simulink model "ART_1G_MMU_SLDRT"  (R2021a)
settings: configuration reference "Normal_SLDRT" (kept outside this file)
undefined symbols (not defined in the file): channel, desired_trajectory_index, group_IP_address, receive_multicast_udp_port_initialize, release_receive_multicast_udp_buffer, release_send_multicast_udp_buffer, send_multicast_udp_data, send_multicast_udp_port_initialize, TRDP_COM_ID_MC2_IDS2MMU, TRDP_COM_ID_MC2_MMU2IDS_POINT, TRDP_COM_ID_MC2_MMU2IDS_SEGMENT, TRDP_CONFIG_MC2_IDS2MMU, TRDP_output, TRDP_SIGNALS_MC2_IDS2MMU, TRDP_SIGNALS_MC2_MMU2IDS_POINT, TRDP_SIGNALS_MC2_MMU2IDS_SEGMENT, UDP_port
libraries: etargetslib x2, simulink x1, sldrtlib x1
settings Model: DataDictionary=ART_1G_MMU.sldd  Creator=xinrui  LastModifiedBy=xinrui
settings ConfigSetRef: SourceName=Normal_SLDRT

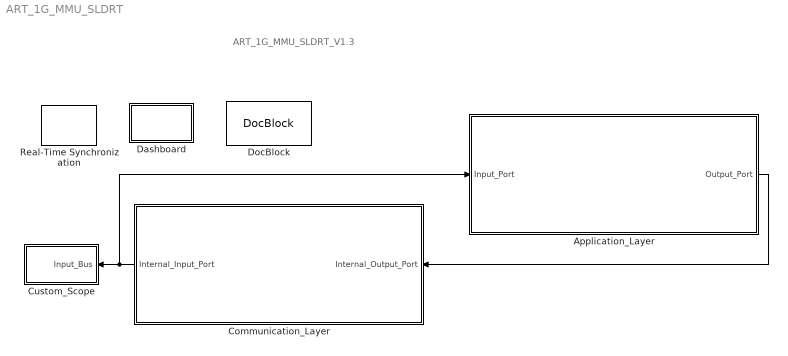
== system ART_1G_MMU_SLDRT ==
  note: ART_1G_MMU_SLDRT_V1.3
  Application_Layer : Subsystem
  Communication_Layer : Subsystem
  Custom_Scope : Subsystem
  Dashboard : Subsystem
  DocBlock : simulink/Model-Wide Utilities/DocBlock  DocumentType=HTML  mask(DocBlock){}
      mask Display:
      | plot([.8 0 0 1 1 .8 .8 1],[1 1 0 0 .8 1 .8 .8]);
      | text(.5,.6,'CHANGELOG','horizontalalignment','center');
      | text(.95,.05,get_param(gcb,'DocumentType'),'verticalalignment','bottom','horizontalalignment','right');
  Real-Time Synchronization : sldrtlib/Real-Time Synchronization  SampleTime=-1  MaxMissedTicks=10  ShowMissedTicks=off  YieldWhenWaiting=off
  wires:
  Application_Layer/1(Output_Port) -> Communication_Layer/1(Internal_Output_Port)
  Communication_Layer/1(Internal_Input_Port) -> Custom_Scope/1(Input_Bus), Application_Layer/1(Input_Port)

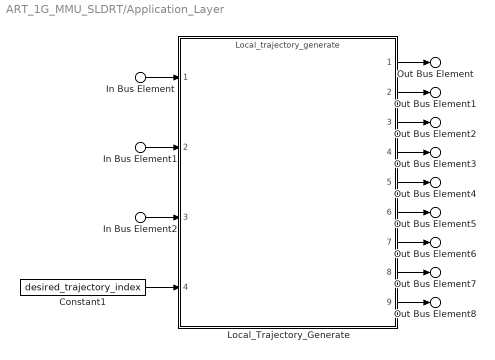
== system ART_1G_MMU_SLDRT/Application_Layer ==
  In Bus Element : Inport  PortName=Input_Port  Element=GNSS_info.ENU_yaw_angle
  In Bus Element1 : Inport  PortName=Input_Port  Element=GNSS_info.ENU_x
  In Bus Element2 : Inport  PortName=Input_Port  Element=GNSS_info.ENU_y
  Constant1 : Constant  Value=desired_trajectory_index  OutDataTypeStr=int8  SampleTime=-1
  Local_Trajectory_Generate : ModelReference  ModelNameDialog=Local_trajectory_generate.slx  SimulationMode=Normal  ModelReferenceVersion=1.197
  Out Bus Element : Outport  PortName=Output_Port  Element=reference_trajectory_info.way_point_number
  Out Bus Element1 : Outport  PortName=Output_Port  Element=reference_trajectory_info.trajectory_yaw_angle
  Out Bus Element2 : Outport  PortName=Output_Port  Element=reference_trajectory_info.trajectory_x
  Out Bus Element3 : Outport  PortName=Output_Port  Element=reference_trajectory_info.trajectory_y
  Out Bus Element4 : Outport  PortName=Output_Port  Element=reference_trajectory_info.trajectory_curvature
  Out Bus Element5 : Outport  PortName=Output_Port  Element=reference_trajectory_info.segment_length
  Out Bus Element6 : Outport  PortName=Output_Port  Element=reference_trajectory_info.segment_ID
  Out Bus Element7 : Outport  PortName=Output_Port  Element=reference_trajectory_info.vision_priority
  Out Bus Element8 : Outport  PortName=Output_Port  Element=reference_trajectory_info.GNSS_priority
  wires:
  In Bus Element/1 -> Local_Trajectory_Generate/1
  In Bus Element1/1 -> Local_Trajectory_Generate/2
  In Bus Element2/1 -> Local_Trajectory_Generate/3
  Constant1/1 -> Local_Trajectory_Generate/4
  Local_Trajectory_Generate/1 -> Out Bus Element/1
  Local_Trajectory_Generate/2 -> Out Bus Element1/1
  Local_Trajectory_Generate/3 -> Out Bus Element2/1
  Local_Trajectory_Generate/4 -> Out Bus Element3/1
  Local_Trajectory_Generate/5 -> Out Bus Element4/1
  Local_Trajectory_Generate/6 -> Out Bus Element5/1
  Local_Trajectory_Generate/7 -> Out Bus Element6/1
  Local_Trajectory_Generate/8 -> Out Bus Element7/1
  Local_Trajectory_Generate/9 -> Out Bus Element8/1

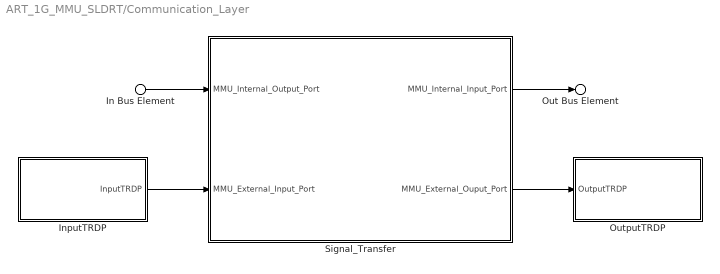
== system ART_1G_MMU_SLDRT/Communication_Layer ==
  In Bus Element : Inport  PortName=Internal_Output_Port
  InputTRDP : Subsystem
  OutputTRDP : Subsystem
  Signal_Transfer : Subsystem
  Out Bus Element : Outport  PortName=Internal_Input_Port
  wires:
  InputTRDP/1(InputTRDP) -> Signal_Transfer/2(MMU_External_Input_Port)
  Signal_Transfer/2(MMU_External_Ouput_Port) -> OutputTRDP/1(OutputTRDP)
  Signal_Transfer/1(MMU_Internal_Input_Port) -> Out Bus Element/1
  In Bus Element/1 -> Signal_Transfer/1(MMU_Internal_Output_Port)

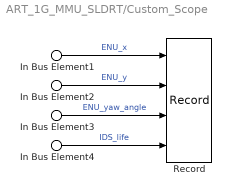
== system ART_1G_MMU_SLDRT/Custom_Scope ==
  In Bus Element4 : Inport  PortName=Input_Bus  Element=GNSS_info.IDS_life
  In Bus Element3 : Inport  PortName=Input_Bus  Element=GNSS_info.ENU_yaw_angle
  In Bus Element1 : Inport  PortName=Input_Bus  Element=GNSS_info.ENU_x
  In Bus Element2 : Inport  PortName=Input_Bus  Element=GNSS_info.ENU_y
  Record : Record  FileSettingsInternal="{\"entries\":[{\"content\":{\"excelSettings\":{\"content\":{},\"type\":\"Streamout.ExcelSettings\"}},\"type\":\"Streamout.FileSettingStorage\",\"uuid\":\"b385ce27-914b-4eb0-ba1e-7ce3f6adea96\"}],\"packageUris\":[\"http://schema.mathworks.com/mf0/streamout_blocks/R2020a\"],\"version\":\"1.0\"}"  SignalsInternal="{\"entries\":[{\"content\":{\"signals\":[{\"content\":{\"blockPath\":[\"ART_1G_MMU_SLDRT/Custom_Scope/Record\"],\"channel\":[],\"dimensions\":[1],\"domain\":\"art_1g_mmu_sldrt/custom_scope/record\",\"lineColor\":\"#fe330a\",\"plots\":[1],\"port\":1,\"sid\":[],\"signalID\":17,\"signalName\":\"ENU_x\"},\"type\":\"RecordBlkView.Signal\",\"uuid\":\"1c878044-c085-469f-83b2-23cc45d2e1f7\"},{\"content\":{\"blockPath\":[\"ART_1G_MMU_SLDRT/Custom_Scope/Record\"],\"channel\":[],\"dimensions\":[1],\"domain\":\"art_1g_mmu_sldrt/custom_scope/record\",\"lineColor\":\"#22b573\",\"plots\":[1],\"port\":2,\"sid\":[],\"signalID\":20,\"signalName\":\"ENU_y\"},\"type\":\"RecordBlkView.Signal\",\"uuid\":\"3e902b27-6836-4cfc-9093-87624b6d09b1\"},{\"content\":{\"blockPath\":[\"ART_1G_MMU_SLDRT/Custom_Scope/Record\"],\"channel\":[],\"dimensions\":[1],\"domain\":\"art_1g_mmu_sldrt/custom_scope/record\",\"lineColor\":\"#0072bd\",\"plots\":[1],\"port\":3,\"sid\":[],\"signalID\":23,\"signalName\":\"ENU_yaw_angle\"},\"type\":\"RecordBlkView.Signal\",\"uuid\":\"fcb5fd97-d04c-438d-9381-11e283686239\"},{\"content\":{\"blockPath\":[\"ART_1G_MMU_SLDRT/Custom_Scope/Record\"],\"channel\":[],\"dimensions\":[1],\"domain\":\"art_1g_mmu_sldrt/custom_scope/record\",\"lineColor\":\"#d95319\",\"plots\":[1],\"port\":4,\"sid\":[],\"signalID\":26,\"signalName\":\"IDS_life\"},\"type\":\"RecordBlkView.Signal\",\"uuid\":\"47ad125d-8b9f-42d6-9a26-871b412a9733\"}]},\"type\":\"RecordBlkView.InputSignals\",\"uuid\":\"3e8808c3-35fa-4291-be64-9e190534e553\"}],\"packageUris\":[\"http://schema.mathworks.com/mf0/streamout_blocks/R2020a\"],\"version\":\"1.0\"}"  VisualizationBindings="{\"sparklinesplugin\":{\"info\":[{\"bindingParametersList\":[],\"subplotID\":1}]}}"
  wires:
  In Bus Element1/1 -> Record/1  "ENU_x"
  In Bus Element2/1 -> Record/2  "ENU_y"
  In Bus Element3/1 -> Record/3  "ENU_yaw_angle"
  In Bus Element4/1 -> Record/4  "IDS_life"

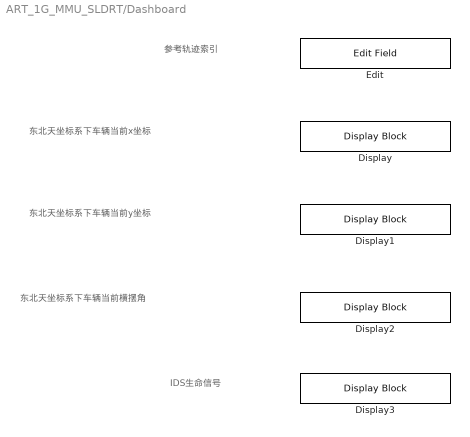
== system ART_1G_MMU_SLDRT/Dashboard ==
  note: 东北天坐标系下车辆当前x坐标
  note: 东北天坐标系下车辆当前y坐标
  note: 东北天坐标系下车辆当前横摆角
  note: IDS生命信号
  note: 参考轨迹索引
  Display{,1..3} (4 alike) : DisplayBlock  Format=short  Transparency=1
  Edit : EditField  LabelPosition=Hide  ShowInitialText=on  Alignment=Center

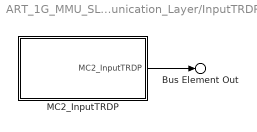
== system ART_1G_MMU_SLDRT/Communication_Layer/InputTRDP ==
  MC2_InputTRDP : Subsystem
  Bus Element Out : Outport  PortName=InputTRDP  Element=MC2_InputTRDP_bus
  wires:
  MC2_InputTRDP/1(MC2_InputTRDP) -> Bus Element Out/1

== system ART_1G_MMU_SLDRT/Communication_Layer/OutputTRDP ==
  Bus Element In1 : Inport  PortName=OutputTRDP  Element=MC2_OutputTRDP_bus
  MC2_OutputTRDP : Subsystem
  wires:
  Bus Element In1/1 -> MC2_OutputTRDP/1(MC2_OutputTRDP)

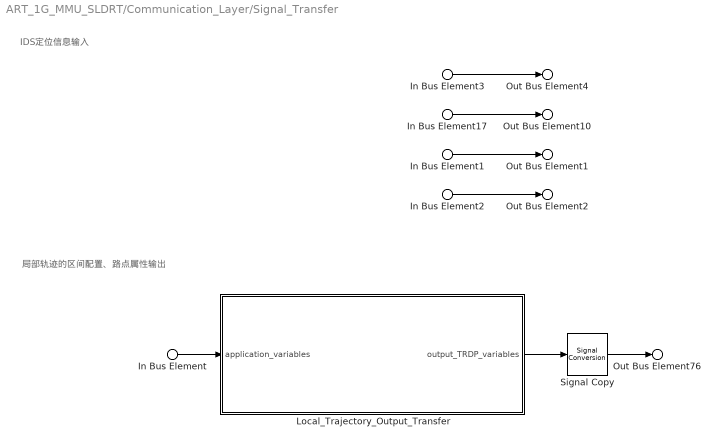
== system ART_1G_MMU_SLDRT/Communication_Layer/Signal_Transfer ==
  note: 局部轨迹的区间配置、路点属性输出
  note: IDS定位信息输入
  In Bus Element : Inport  PortName=MMU_Internal_Output_Port
  In Bus Element2 : Inport  Port=2  PortName=MMU_External_Input_Port  Element=MC2_InputTRDP_bus.MC2_IDS2MMU_bus.ENU_yaw_angle
  In Bus Element17 : Inport  Port=2  PortName=MMU_External_Input_Port  Element=MC2_InputTRDP_bus.MC2_IDS2MMU_bus.ENU_x
  In Bus Element1 : Inport  Port=2  PortName=MMU_External_Input_Port  Element=MC2_InputTRDP_bus.MC2_IDS2MMU_bus.ENU_y
  In Bus Element3 : Inport  Port=2  PortName=MMU_External_Input_Port  Element=MC2_InputTRDP_bus.MC2_IDS2MMU_bus.IDS_life
  Local_Trajectory_Output_Transfer : MATLAB Function  TreatAsAtomicUnit=on
  Signal Copy : SignalConversion  ConversionOutput=Virtual bus  OverrideOpt=off
  Out Bus Element4 : Outport  PortName=MMU_Internal_Input_Port  Element=GNSS_info.IDS_life
  Out Bus Element2 : Outport  PortName=MMU_Internal_Input_Port  Element=GNSS_info.ENU_yaw_angle
  Out Bus Element10 : Outport  PortName=MMU_Internal_Input_Port  Element=GNSS_info.ENU_x
  Out Bus Element1 : Outport  PortName=MMU_Internal_Input_Port  Element=GNSS_info.ENU_y
  Out Bus Element76 : Outport  Port=2  PortName=MMU_External_Ouput_Port  Element=MC2_OutputTRDP_bus
  wires:
  In Bus Element17/1 -> Out Bus Element10/1
  In Bus Element1/1 -> Out Bus Element1/1
  In Bus Element2/1 -> Out Bus Element2/1
  In Bus Element/1 -> Local_Trajectory_Output_Transfer/1(application_variables)
  Local_Trajectory_Output_Transfer/1(output_TRDP_variables) -> Signal Copy/1
  Signal Copy/1 -> Out Bus Element76/1
  In Bus Element3/1 -> Out Bus Element4/1

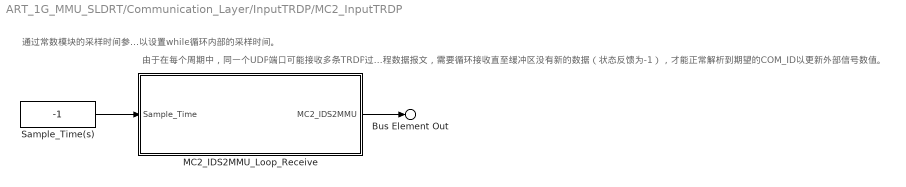
== system ART_1G_MMU_SLDRT/Communication_Layer/InputTRDP/MC2_InputTRDP ==
  note: 通过常数模块的采样时间参数可以设置while循环内部的采样时间。
  note: 由于在每个周期中，同一个UDP端口可能接收多条TRDP过程数据报文，需要循环接收直至缓冲区没有新的数据（状态反馈为-1），才能正常解析到期望的COM_ID以更新外部信号数值。
  MC2_IDS2MMU_Loop_Receive : Subsystem  TreatAsAtomicUnit=on
  Sample_Time(s) : Constant  Value=-1  SampleTime=-1
  Bus Element Out : Outport  PortName=MC2_InputTRDP  Element=MC2_IDS2MMU_bus
  wires:
  MC2_IDS2MMU_Loop_Receive/1(MC2_IDS2MMU) -> Bus Element Out/1
  Sample_Time(s)/1 -> MC2_IDS2MMU_Loop_Receive/1(Sample_Time)

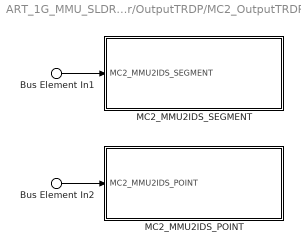
== system ART_1G_MMU_SLDRT/Communication_Layer/OutputTRDP/MC2_OutputTRDP ==
  Bus Element In1 : Inport  PortName=MC2_OutputTRDP  Element=MC2_MMU2IDS_SEGMENT_bus
  Bus Element In2 : Inport  PortName=MC2_OutputTRDP  Element=MC2_MMU2IDS_POINT_bus
  MC2_MMU2IDS_POINT : Subsystem
  MC2_MMU2IDS_SEGMENT : Subsystem
  wires:
  Bus Element In1/1 -> MC2_MMU2IDS_SEGMENT/1(MC2_MMU2IDS_SEGMENT)
  Bus Element In2/1 -> MC2_MMU2IDS_POINT/1(MC2_MMU2IDS_POINT)

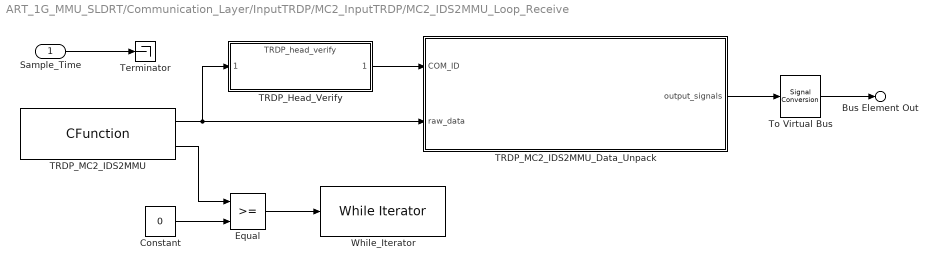
== system ART_1G_MMU_SLDRT/Communication_Layer/InputTRDP/MC2_InputTRDP/MC2_IDS2MMU_Loop_Receive ==
  Sample_Time : Inport
  Constant : Constant  Value=0  OutDataTypeStr=int32
  Equal : RelationalOperator  OutDataTypeStr=boolean  RndMeth=Simplest
  TRDP_Head_Verify : ModelReference  ModelNameDialog=TRDP_head_verify  SimulationMode=Normal  ModelReferenceVersion=1.48
  TRDP_MC2_IDS2MMU : CFunction  OutputCode=|  TerminateCode=release_receive_multicast_udp_buffer(channel);  StartCode=receive_multicast_udp_port_initialize(group_IP_address, UDP_port, channel);  group_IP_address=uint8(['239.255.3.101',0])  UDP_port=int32(17224)  channel=int32(0)
      | int index;
      | uint8_T *receive_buffer;
      | data_length = receive_multicast_udp_data(channel);
      | receive_buffer = get_multicast_udp_data(channel);
      | for(index = 0; index < RECEIVE_MULTICAST_UDP_BUFFER_SIZE; index++)
      | {
      |     TRDP_input[index] = receive_buffer[index];
      | }
  TRDP_MC2_IDS2MMU_Data_Unpack : MATLAB Function  TreatAsAtomicUnit=on
  Terminator : Terminator
  To Virtual Bus : SignalConversion  ConversionOutput=Virtual bus  OverrideOpt=off
  While_Iterator : WhileIterator  MaxIters=-1  WhileBlockType=do-while
  Bus Element Out : Outport  PortName=MC2_IDS2MMU
  wires:
  Equal/1 -> While_Iterator/1
  Sample_Time/1 -> Terminator/1
  To Virtual Bus/1 -> Bus Element Out/1
  TRDP_MC2_IDS2MMU_Data_Unpack/1(output_signals) -> To Virtual Bus/1
  TRDP_MC2_IDS2MMU/1 -> TRDP_Head_Verify/1, TRDP_MC2_IDS2MMU_Data_Unpack/2(raw_data)
  Constant/1 -> Equal/2
  TRDP_MC2_IDS2MMU/2 -> Equal/1
  TRDP_Head_Verify/1 -> TRDP_MC2_IDS2MMU_Data_Unpack/1(COM_ID)

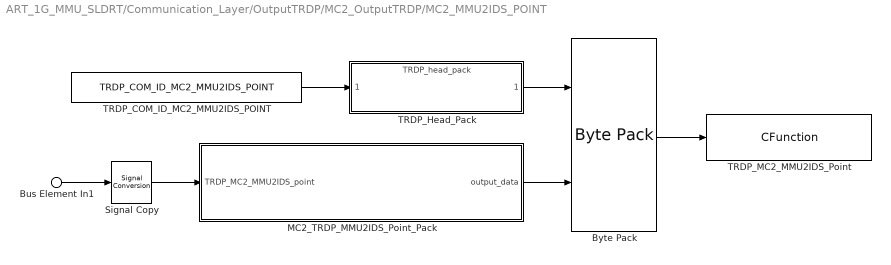
== system ART_1G_MMU_SLDRT/Communication_Layer/OutputTRDP/MC2_OutputTRDP/MC2_MMU2IDS_POINT ==
  Bus Element In1 : Inport  PortName=MC2_MMU2IDS_POINT
  Byte Pack : etargetslib/Byte Pack  datatypes={'uint8', 'uint8'}  byteAlign=1
  MC2_TRDP_MMU2IDS_Point_Pack : MATLAB Function  TreatAsAtomicUnit=on
  Signal Copy : SignalConversion  ConversionOutput=Nonvirtual bus  OutDataTypeStr=Bus: MC2_MMU2IDS_POINT  OverrideOpt=off
  TRDP_COM_ID_MC2_MMU2IDS_POINT : Constant  Value=TRDP_COM_ID_MC2_MMU2IDS_POINT  OutDataTypeStr=uint32  SampleTime=-1
  TRDP_Head_Pack : ModelReference  ModelNameDialog=TRDP_head_pack  SimulationMode=Normal  ModelReferenceVersion=1.47
  TRDP_MC2_MMU2IDS_Point : CFunction  OutputCode=send_multicast_udp_data(TRDP_output, channel);  TerminateCode=release_send_multicast_udp_buffer(channel);  StartCode=send_multicast_udp_port_initialize(group_IP_address, UDP_port, channel);  group_IP_address=uint8(['239.255.3.101',0])  UDP_port=int32(17224)  channel=int32(0)
  wires:
  MC2_TRDP_MMU2IDS_Point_Pack/1(output_data) -> Byte Pack/2
  TRDP_COM_ID_MC2_MMU2IDS_POINT/1 -> TRDP_Head_Pack/1
  TRDP_Head_Pack/1 -> Byte Pack/1
  Byte Pack/1 -> TRDP_MC2_MMU2IDS_Point/1
  Bus Element In1/1 -> Signal Copy/1
  Signal Copy/1 -> MC2_TRDP_MMU2IDS_Point_Pack/1(TRDP_MC2_MMU2IDS_point)

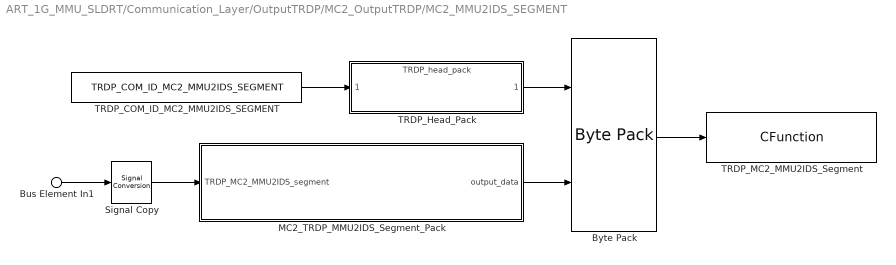
== system ART_1G_MMU_SLDRT/Communication_Layer/OutputTRDP/MC2_OutputTRDP/MC2_MMU2IDS_SEGMENT ==
  Bus Element In1 : Inport  PortName=MC2_MMU2IDS_SEGMENT
  Byte Pack : etargetslib/Byte Pack  datatypes={'uint8', 'uint8'}  byteAlign=1
  MC2_TRDP_MMU2IDS_Segment_Pack : MATLAB Function  TreatAsAtomicUnit=on
  Signal Copy : SignalConversion  ConversionOutput=Nonvirtual bus  OutDataTypeStr=Bus: MC2_MMU2IDS_SEGMENT  OverrideOpt=off
  TRDP_COM_ID_MC2_MMU2IDS_SEGMENT : Constant  Value=TRDP_COM_ID_MC2_MMU2IDS_SEGMENT  OutDataTypeStr=uint32  SampleTime=-1
  TRDP_Head_Pack : ModelReference  ModelNameDialog=TRDP_head_pack  SimulationMode=Normal  ModelReferenceVersion=1.47
  TRDP_MC2_MMU2IDS_Segment : CFunction  OutputCode=send_multicast_udp_data(TRDP_output, channel);  TerminateCode=release_send_multicast_udp_buffer(channel);  StartCode=send_multicast_udp_port_initialize(group_IP_address, UDP_port, channel);  group_IP_address=uint8(['239.255.3.101',0])  UDP_port=int32(17224)  channel=int32(0)
  wires:
  Byte Pack/1 -> TRDP_MC2_MMU2IDS_Segment/1
  TRDP_Head_Pack/1 -> Byte Pack/1
  TRDP_COM_ID_MC2_MMU2IDS_SEGMENT/1 -> TRDP_Head_Pack/1
  MC2_TRDP_MMU2IDS_Segment_Pack/1(output_data) -> Byte Pack/2
  Bus Element In1/1 -> Signal Copy/1
  Signal Copy/1 -> MC2_TRDP_MMU2IDS_Segment_Pack/1(TRDP_MC2_MMU2IDS_segment)

== matlab function ART_1G_MMU_SLDRT/Communication_Layer/OutputTRDP/MC2_OutputTRDP/MC2_MMU2IDS_POINT/MC2_TRDP_MMU2IDS_Point_Pack ==
  data: TRDP_MC2_MMU2IDS_point input Bus: MC2_MMU2IDS_POINT size=1; output_data output uint8 size=1000; TRDP_CONFIG_MC2_MMU2IDS_POINT parameter Bus: CONFIG_MC2_MMU2IDS_POINT size=1
% TRDP数据打包
function output_data = MC2_TRDP_MMU2IDS_point_pack(TRDP_MC2_MMU2IDS_point, ...
    TRDP_CONFIG_MC2_MMU2IDS_POINT)
%   1.输入参数：
%       (1)TRDP_MC2_MMU2IDS_point           TRDP_MC2_MMU2IDS_point信号结构体，匹配MC2_MMU2IDS_POINT总线类型
%       (2)TRDP_CONFIG_MC2_MMU2IDS_POINT    MC2端MMU发给IDS的路点属性TRDP数据打包配置参数，Parameter，数据字典中的一个结构体
%   2.输出参数：
%       (1)output_data                      输出TRDP数据，1000×1的uint8向量

%% 输出信号编码打包
output_data = TRDP_output_data_pack(1000, TRDP_CONFIG_MC2_MMU2IDS_POINT, ...
    TRDP_MC2_MMU2IDS_point);

end

== matlab function ART_1G_MMU_SLDRT/Communication_Layer/Signal_Transfer/Local_Trajectory_Output_Transfer ==
  data: application_variables input Bus: ApplicationBus size=1; output_TRDP_variables output Bus: MC2_OutputTRDP size=1; TRDP_SIGNALS_MC2_MMU2IDS_SEGMENT parameter Bus: MC2_MMU2IDS_SEGMENT size=1; TRDP_SIGNALS_MC2_MMU2IDS_POINT parameter Bus: MC2_MMU2IDS_POINT size=1
% 局部轨迹输出转发到TRDP变量集
function output_TRDP_variables = Local_trajectory_output_transfer(application_variables, ...
    TRDP_SIGNALS_MC2_MMU2IDS_SEGMENT, TRDP_SIGNALS_MC2_MMU2IDS_POINT)
%   1.输入参数：
%       (1)application_variables    应用层的变量集
%   2.输出参数：
%       (1)output_TRDP_variables    输出TRDP变量集，匹配MC2_IDS2MMU总线类型

%% 初始化
output_TRDP_variables.MC2_MMU2IDS_SEGMENT_bus = TRDP_SIGNALS_MC2_MMU2IDS_SEGMENT;
output_TRDP_variables.MC2_MMU2IDS_POINT_bus = TRDP_SIGNALS_MC2_MMU2IDS_POINT;

%% 获取输出结构体的成员名称列表
segment_names = fieldnames(TRDP_SIGNALS_MC2_MMU2IDS_SEGMENT);
point_names = fieldnames(output_TRDP_variables.MC2_MMU2IDS_POINT_bus);

%% 局部轨迹区间配置变量转发到TRDP变量集
% 生命信号转发IDS的生命信号，便于后续排查通信问题
output_TRDP_variables.MC2_MMU2IDS_SEGMENT_bus.segment_data_life = ...
    application_variables.GNSS_info.IDS_life;

% 有效区间数量是应用变量集里的轨迹区间代号中不重复的非零数值数量
original_segment_ID = application_variables.reference_trajectory_info.segment_ID(...
    0 < application_variables.reference_trajectory_info.segment_ID);
[unique_segment_ID, original_index, ~] = unique(original_segment_ID);
output_TRDP_variables.MC2_MMU2IDS_SEGMENT_bus.segment_number = length(unique_segment_ID);

% 遍历应用变量集里的全部有效区间，转发配置参数
if 0 >= length(unique_segment_ID)
    return;
end
for index1 = 1 : length(unique_segment_ID)
    
    % 拼接指定区间配置结构体成员名称
    temp_segment_ID_name = sprintf('segment_%u_ID', uint32(index1));
    temp_segment_way_point_interval_name = sprintf('segment_%u_way_point_interval', ...
        uint32(index1));
    temp_segment_vision_priority_name = sprintf('segment_%u_vision_priority', ...
        uint32(index1));
    temp_segment_GNSS_priority_name = sprintf('segment_%u_GNSS_priority', ...
        uint32(index1));

    % 遍历TRDP区间配置变量结构体，转发配置参数
    for index2 = 1 : length(segment_names)
        if strcmp(segment_names{index2}, temp_segment_ID_name)
            output_TRDP_variables.MC2_MMU2IDS_SEGMENT_bus.(segment_names{index2}) = ...
                double(unique_segment_ID(index1));
        end
        if strcmp(segment_names{index2}, temp_segment_way_point_interval_name)
            output_TRDP_variables.MC2_MMU2IDS_SEGMENT_bus.(segment_names{index2}) = ...
                application_variables.reference_trajectory_info.segment_length(...
                original_index(index1));
        end
        if strcmp(segment_names{index2}, temp_segment_vision_priority_name)
            output_TRDP_variables.MC2_MMU2IDS_SEGMENT_bus.(segment_names{index2}) = ...
                double(application_variables.reference_trajectory_info.vision_priority(...
                original_index(index1)));
        end
        if strcmp(segment_names{index2}, temp_segment_GNSS_priority_name)
            output_TRDP_variables.MC2_MMU2IDS_SEGMENT_bus.(segment_names{index2}) = ...
                double(application_variables.reference_trajectory_info.GNSS_priority(...
                original_index(index1)));
        end
    end
    
end

%% 局部轨迹路点属性变量转发到TRDP变量集
% 生命信号转发IDS的生命信号，便于后续排查通信问题
output_TRDP_variables.MC2_MMU2IDS_POINT_bus.way_point_data_life = ...
    application_variables.GNSS_info.IDS_life;

% 直接转发应用变量集里的有效路点数量
output_TRDP_variables.MC2_MMU2IDS_POINT_bus.way_point_number = ...
    double(application_variables.reference_trajectory_info.way_point_number);

% 遍历应用变量集里的全部有效路点，转发属性参数
if 0 >= application_variables.reference_trajectory_info.way_point_number
    return;
end
for index1 = 1 : application_variables.reference_trajectory_info.way_point_number
    
    % 拼接指定路点属性结构体成员名称
    temp_point_yaw_angle_name = sprintf('way_point_%u_yaw_angle', uint32(index1));
    temp_point_x_name = sprintf('way_point_%u_x', uint32(index1));
    temp_point_y_name = sprintf('way_point_%u_y', uint32(index1));
    temp_point_curvature_name = sprintf('way_point_%u_curvature', uint32(index1));

    % 遍历TRDP路点属性变量结构体，转发属性参数
    for index2 = 1 : length(point_names)
        if strcmp(point_names{index2}, temp_point_yaw_angle_name)
            output_TRDP_variables.MC2_MMU2IDS_POINT_bus.(point_names{index2}) = ...
                application_variables.reference_trajectory_info.trajectory_yaw_angle(index1);
        end
        if strcmp(point_names{index2}, temp_point_x_name)
            output_TRDP_variables.MC2_MMU2IDS_POINT_bus.(point_names{index2}) = ...
                application_variables.reference_trajectory_info.trajectory_x(index1);
        end
        if strcmp(point_names{index2}, temp_point_y_name)
            output_TRDP_variables.MC2_MMU2IDS_POINT_bus.(point_names{index2}) = ...
                application_variables.reference_trajectory_info.trajectory_y(index1);
        end
        if strcmp(point_names{index2}, temp_point_curvature_name)
            output_TRDP_variables.MC2_MMU2IDS_POINT_bus.(point_names{index2}) = ...
                application_variables.reference_trajectory_info.trajectory_curvature(index1);
        end
    end
    
end

end

== matlab function ART_1G_MMU_SLDRT/Communication_Layer/InputTRDP/MC2_InputTRDP/MC2_IDS2MMU_Loop_Receive/TRDP_MC2_IDS2MMU_Data_Unpack ==
  data: COM_ID input uint32 size=1; raw_data input uint8 size=1040; output_signals output Bus: MC2_IDS2MMU size=1; TRDP_CONFIG_MC2_IDS2MMU parameter Bus: CONFIG_MC2_IDS2MMU size=1; TRDP_SIGNALS_MC2_IDS2MMU parameter Bus: MC2_IDS2MMU size=1; TRDP_COM_ID_MC2_IDS2MMU parameter double size=1
% TRDP数据解包
function output_signals = TRDP_MC2_IDS2MMU_data_unpack(COM_ID, raw_data, ...
    TRDP_CONFIG_MC2_IDS2MMU, TRDP_SIGNALS_MC2_IDS2MMU, TRDP_COM_ID_MC2_IDS2MMU)
%   1.输入参数：
%       (1)COM_ID                      TRDP通信索引，1×1的uint32向量
%       (2)raw_data                    TRDP原始数据，1040×1的uint8向量
%       (3)TRDP_CONFIG_MC2_IDS2MMU     MC2端IDS发给MMU的TRDP原始数据解析配置参数，Parameter，数据字典中的一个结构体
%       (4)TRDP_SIGNALS_MC2_IDS2MMU    MC2端IDS发给MMU的TRDP信号结构初始值，Parameter，数据字典中的一个结构体
%       (5)TRDP_COM_ID_MC2_IDS2MMU     MC2端IDS发给MMU的TRDP过程数据COM ID，Parameter，数据字典中的一个Parameter变量
%   2.输出参数：
%       (1)output_signals              输出信号结构体，匹配MC2_IDS2MMU总线类型

%% 静态变量声明及初始化
% IDS2MMU信号结构体，用于存储上周期IDS相关信号数值
persistent TRDP_IDS2MMU_signals;
if isempty(TRDP_IDS2MMU_signals)
   TRDP_IDS2MMU_signals = TRDP_SIGNALS_MC2_IDS2MMU;
end

%% 检查COM_ID和数据长度，与预期匹配才则将后1000个字节解析为IDS2MMU数据
if TRDP_COM_ID_MC2_IDS2MMU == COM_ID && 1040 == length(raw_data)
    TRDP_IDS2MMU_signals = TRDP_input_data_parse(raw_data(41 : 1040), ...
        TRDP_CONFIG_MC2_IDS2MMU, TRDP_IDS2MMU_signals);
end

%% 输出信号赋值
output_signals = TRDP_IDS2MMU_signals;

end

== matlab function ART_1G_MMU_SLDRT/Communication_Layer/OutputTRDP/MC2_OutputTRDP/MC2_MMU2IDS_SEGMENT/MC2_TRDP_MMU2IDS_Segment_Pack ==
  data: TRDP_MC2_MMU2IDS_segment input Bus: MC2_MMU2IDS_SEGMENT size=1; output_data output uint8 size=1000; TRDP_CONFIG_MC2_MMU2IDS_SEGMENT parameter Bus: CONFIG_MC2_MMU2IDS_SEGMENT size=1
% TRDP数据打包
function output_data = MC2_TRDP_MMU2IDS_segment_pack(TRDP_MC2_MMU2IDS_segment, ...
    TRDP_CONFIG_MC2_MMU2IDS_SEGMENT)
%   1.输入参数：
%       (1)TRDP_MC2_MMU2IDS_segment           TRDP_MC2_MMU2IDS_segment信号结构体，匹配MC2_MMU2IDS_SEGMENT总线类型
%       (2)TRDP_CONFIG_MC2_MMU2IDS_SEGMENT    MC2端MMU发给IDS的区间配置TRDP数据打包配置参数，Parameter，数据字典中的一个结构体
%   2.输出参数：
%       (1)output_data                        输出TRDP数据，1000×1的uint8向量

%% 输出信号编码打包
output_data = TRDP_output_data_pack(1000, TRDP_CONFIG_MC2_MMU2IDS_SEGMENT, ...
    TRDP_MC2_MMU2IDS_segment);

end
